simulink model "Sim2Twin_controlsystem_pos_Discrete"  (R2024b)
settings: Solver=FixedStepAuto  StartTime=0.0  StopTime=10.0  FixedStep=0.001  RelTol=1e-3
undefined symbols (not defined in the file): DiscIntNeverNeededParam, dspblkCoreblockFVToolHelper, gcbh
libraries: simulink x1
settings Model: Creator=Emila  LastModifiedBy=Are-Laptop
settings ConfigComp: PLC_OutputDir=XML  PLC_TargetIDE=twincat3  PLC_MultiTBSigbuilderTimeRange=off  PLC_FoldFBCallOutputVar=off  PLC_RemoveUnusedSSMethodCallArguments=off  PLC_UseCallOutputArgSyntax=off  PLC_EnableUnsignedAndDoubleTypes=off  PLC_EnableUDTSplitting=off  PLC_MaxFieldsInUDT=500  PLC_InlineEnumCastFunction=off

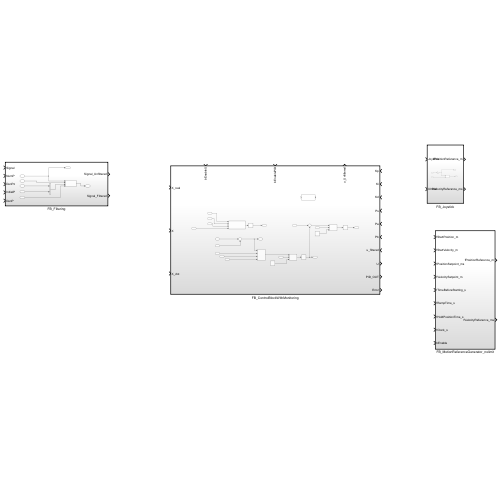
[thumbnail: Simulink's stored preview of the top-level diagram]
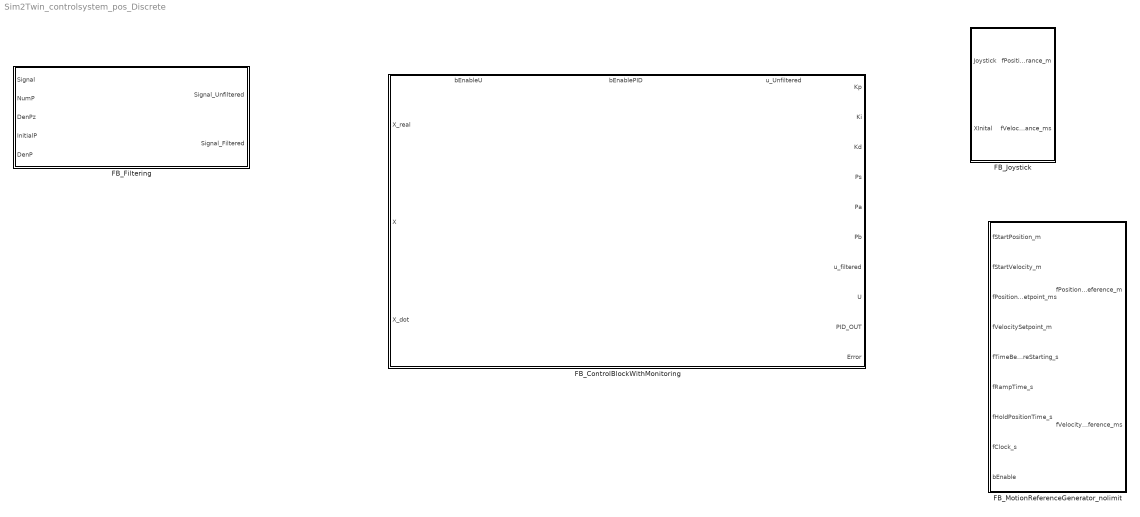
== system Sim2Twin_controlsystem_pos_Discrete ==
  FB_ControlBlockWithMonitoring : Subsystem  TreatAsAtomicUnit=on
      settings: PortSchema="{\"entries\":[{\"content\":{\"sides\":[{\"content\":{\"connectorIds\":[\"In1\",\"In2\",\"In3\"]},\"type\":\"ConnectorPlacement.EquallySpacedRectSide\",\"uuid\":\"e7dc98bc-0c39-42fc-9d44-5c528a861935\"},{\"content\":{\"connectorIds\":[\"In6\",\"In7\",\"In8\",\"In9\",\"In10\",\"In11\",\"In12\",\"Out1\",\"Out2\",\"Out3\"],\"side\":\"RIGHT\"},\"type\":\"ConnectorPlacement.EquallySpacedRectSide\",\"uuid\":\"7a7fb2e4-7f4e-4840-80a8-3a9723ecfbf6\"},{\"content\":{\"connectorIds\":[\"In4\",\"In5\",\"Out4\"],\"side\":\"TOP\"},\"type\":\"ConnectorPlacement.EquallySpacedRectSide\",\"uuid\":\"8314552e-40ce-493a-a910-ea6a3ee6c4fc\"},{\"content\":{\"side\":\"BOTTOM\"},\"type\":\"ConnectorPlacement.EquallySpacedRectSide\",\"uuid\":\"f3f01719-ff93-4fec-8599-54303ea6e608\"}]},\"type\":\"ConnectorPlacement.EquallySpacedConnector\",\"uuid\":\"904788e7-187d-4514-a00a-56ca1dbc298c\"}],\"packageUris\":[\"http://schema.mathworks.com/mf0/Connector/R2020b\"],\"version\":\"1.0\"}"
  FB_Filtering : Subsystem  TreatAsAtomicUnit=on
  FB_Joystick : Subsystem  TreatAsAtomicUnit=on
  FB_MotionReferenceGenerator_nolimit : Subsystem  TreatAsAtomicUnit=on  VariantControl=Ramp_Profile

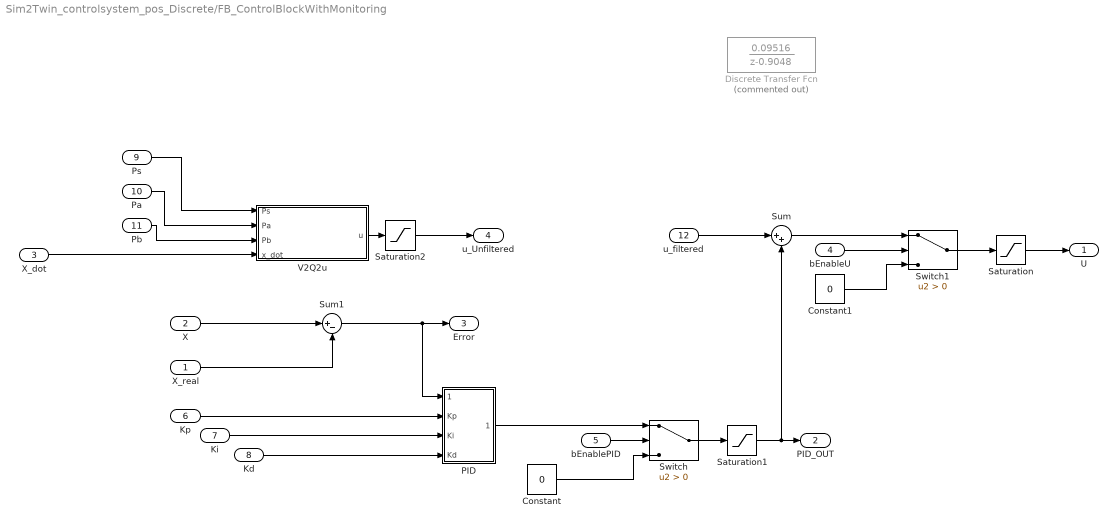
== system Sim2Twin_controlsystem_pos_Discrete/FB_ControlBlockWithMonitoring ==
  X_real : Inport
  X : Inport  Port=2
  X_dot : Inport  Port=3
  bEnableU : Inport  Port=4  OutDataTypeStr=boolean
  bEnablePID : Inport  Port=5  OutDataTypeStr=boolean
  Kp : Inport  Port=6
  Ki : Inport  Port=7
  Kd : Inport  Port=8
  Ps : Inport  Port=9
  Pa : Inport  Port=10
  Pb : Inport  Port=11
  u_filtered : Inport  Port=12
  Constant : Constant  Value=0
  Constant1 : Constant  Value=0
  Discrete Transfer Fcn : DiscreteTransferFcn  Commented=on  LoadFcn=dspblkCoreblockFVToolHelper(gcbh,'load');  Numerator=[0.09516]  Denominator=[1 -0.9048]
      settings: CopyFcn=dspblkCoreblockFVToolHelper(gcbh,'copy');  DeleteFcn=dspblkCoreblockFVToolHelper(gcbh,'close');  ModelCloseFcn=dspblkCoreblockFVToolHelper(gcbh,'close');  PreSaveFcn=dspblkCoreblockFVToolHelper(gcbh,'presave');  PostSaveFcn=dspblkCoreblockFVToolHelper(gcbh,'postsave');  CloseFcn=dspblkCoreblockFVToolHelper(gcbh,'close');
  PID : Subsystem
  Saturation : Saturate  UpperLimit=1  LowerLimit=-1
  Saturation1 : Saturate  UpperLimit=1  LowerLimit=-1
  Saturation2 : Saturate  UpperLimit=1  LowerLimit=-1
  Sum : Sum  Inputs=|++
  Sum1 : Sum  Inputs=|+-
  Switch : Switch  Criteria=u2 > Threshold  SaturateOnIntegerOverflow=off  InputSameDT=off
  Switch1 : Switch  Criteria=u2 > Threshold  SaturateOnIntegerOverflow=off  InputSameDT=off
  V2Q2u : MATLAB Function  TreatAsAtomicUnit=on
  U : Outport
  PID_OUT : Outport  Port=2
  Error : Outport  Port=3
  u_Unfiltered : Outport  Port=4
  wires:
  X_real/1 -> Sum1/2
  Sum1/1 -> Error/1, PID/1(PID_IN)
  V2Q2u/1(u) -> Saturation2/1
  X_dot/1 -> V2Q2u/4(x_dot)
  X/1 -> Sum1/1
  Switch/1 -> Saturation1/1
  PID/1(PID_OUT) -> Switch/1
  Switch1/1 -> Saturation/1
  Sum/1 -> Switch1/1
  bEnableU/1 -> Switch1/2
  bEnablePID/1 -> Switch/2
  Constant/1 -> Switch/3
  Constant1/1 -> Switch1/3
  Kp/1 -> PID/2(Kp)
  Ki/1 -> PID/3(Ki)
  Kd/1 -> PID/4(Kd)
  Saturation/1 -> U/1
  Saturation1/1 -> PID_OUT/1, Sum/2
  Saturation2/1 -> u_Unfiltered/1
  Pb/1 -> V2Q2u/3(Pb)
  Pa/1 -> V2Q2u/2(Pa)
  Ps/1 -> V2Q2u/1(Ps)
  u_filtered/1 -> Sum/1

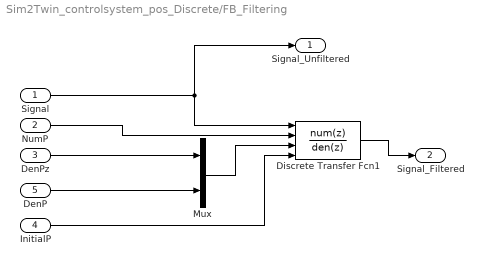
== system Sim2Twin_controlsystem_pos_Discrete/FB_Filtering ==
  Signal : Inport
  NumP : Inport  Port=2
  DenPz : Inport  Port=3
  InitialP : Inport  Port=4
  DenP : Inport  Port=5
  Discrete Transfer Fcn1 : DiscreteTransferFcn  LoadFcn=dspblkCoreblockFVToolHelper(gcbh,'load');  NumeratorSource=Input port  Numerator=[0.003137]  DenominatorSource=Input port  Denominator=[1 -0.9969]  InitialStatesSource=Input port  a0EqualsOne=on
      settings: CopyFcn=dspblkCoreblockFVToolHelper(gcbh,'copy');  DeleteFcn=dspblkCoreblockFVToolHelper(gcbh,'close');  ModelCloseFcn=dspblkCoreblockFVToolHelper(gcbh,'close');  PreSaveFcn=dspblkCoreblockFVToolHelper(gcbh,'presave');  PostSaveFcn=dspblkCoreblockFVToolHelper(gcbh,'postsave');  CloseFcn=dspblkCoreblockFVToolHelper(gcbh,'close');  InputPortMap=u0,p1,p3,p5
  Mux : Mux  Inputs=2
  Signal_Unfiltered : Outport
  Signal_Filtered : Outport  Port=2
  wires:
  InitialP/1 -> Discrete Transfer Fcn1/4
  DenP/1 -> Mux/2
  NumP/1 -> Discrete Transfer Fcn1/2
  DenPz/1 -> Mux/1
  Signal/1 -> Discrete Transfer Fcn1/1, Signal_Unfiltered/1
  Discrete Transfer Fcn1/1 -> Signal_Filtered/1
  Mux/1 -> Discrete Transfer Fcn1/3

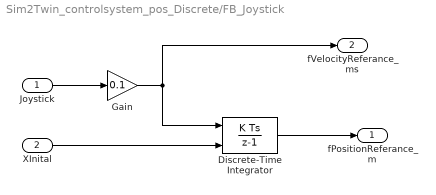
== system Sim2Twin_controlsystem_pos_Discrete/FB_Joystick ==
  Joystick : Inport
  XInital : Inport  Port=2
  Discrete-Time Integrator : DiscreteIntegrator  InitialConditionSource=external  SampleTime=-1  LimitOutput=on  UpperSaturationLimit=0.45  LowerSaturationLimit=0  ICPrevOutput=DiscIntNeverNeededParam  ICPrevScaledInput=DiscIntNeverNeededParam
  Gain : Gain  Gain=0.1
  fPositionReferance_m : Outport
  fVelocityReferance_ms : Outport  Port=2
  wires:
  Joystick/1 -> Gain/1
  Gain/1 -> Discrete-Time Integrator/1, fVelocityReferance_ms/1
  Discrete-Time Integrator/1 -> fPositionReferance_m/1
  XInital/1 -> Discrete-Time Integrator/2

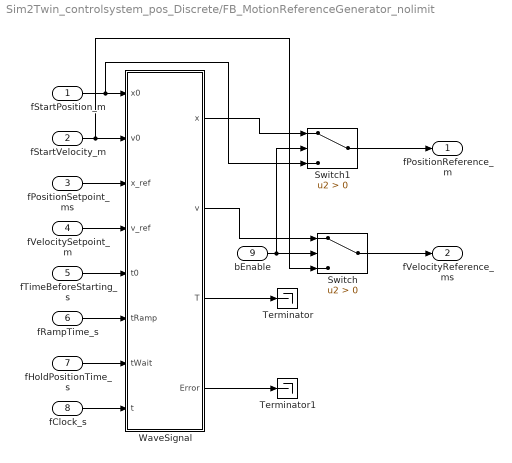
== system Sim2Twin_controlsystem_pos_Discrete/FB_MotionReferenceGenerator_nolimit ==
  fStartPosition_m : Inport
  fStartVelocity_m : Inport  Port=2
  fPositionSetpoint_ms : Inport  Port=3
  fVelocitySetpoint_m : Inport  Port=4
  fTimeBeforeStarting_s : Inport  Port=5
  fRampTime_s : Inport  Port=6
  fHoldPositionTime_s : Inport  Port=7
  fClock_s : Inport  Port=8
  bEnable : Inport  Port=9  OutDataTypeStr=boolean
  Switch : Switch  Criteria=u2 > Threshold  SaturateOnIntegerOverflow=off  InputSameDT=off
  Switch1 : Switch  Criteria=u2 > Threshold  SaturateOnIntegerOverflow=off  InputSameDT=off
  Terminator : Terminator
  Terminator1 : Terminator
  WaveSignal : MATLAB Function  TreatAsAtomicUnit=on
  fPositionReference_m : Outport  VectorParamsAs1DForOutWhenUnconnected=off
  fVelocityReference_ms : Outport  Port=2  VectorParamsAs1DForOutWhenUnconnected=off
  wires:
  fClock_s/1 -> WaveSignal/8(t)
  fTimeBeforeStarting_s/1 -> WaveSignal/5(t0)
  fPositionSetpoint_ms/1 -> WaveSignal/3(x_ref)
  fHoldPositionTime_s/1 -> WaveSignal/7(tWait)
  fVelocitySetpoint_m/1 -> WaveSignal/4(v_ref)
  WaveSignal/3(T) -> Terminator/1
  fRampTime_s/1 -> WaveSignal/6(tRamp)
  WaveSignal/4(Error) -> Terminator1/1
  WaveSignal/2(v) -> Switch/1
  fStartPosition_m/1 -> Switch1/3, WaveSignal/1(x0)
  Switch/1 -> fVelocityReference_ms/1
  bEnable/1 -> Switch1/2, Switch/2
  Switch1/1 -> fPositionReference_m/1
  WaveSignal/1(x) -> Switch1/1
  fStartVelocity_m/1 -> WaveSignal/2(v0), Switch/3

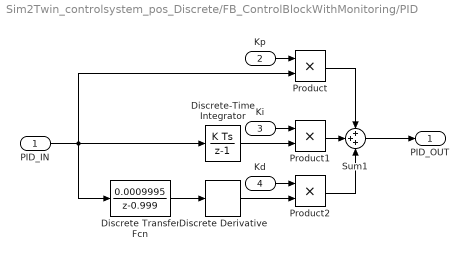
== system Sim2Twin_controlsystem_pos_Discrete/FB_ControlBlockWithMonitoring/PID ==
  PID_IN : Inport
  Kp : Inport  Port=2
  Ki : Inport  Port=3
  Kd : Inport  Port=4
  Discrete Transfer Fcn : DiscreteTransferFcn  LoadFcn=dspblkCoreblockFVToolHelper(gcbh,'load');  Numerator=[0.0009995]  Denominator=[1 -0.999]
      settings: CopyFcn=dspblkCoreblockFVToolHelper(gcbh,'copy');  DeleteFcn=dspblkCoreblockFVToolHelper(gcbh,'close');  ModelCloseFcn=dspblkCoreblockFVToolHelper(gcbh,'close');  PreSaveFcn=dspblkCoreblockFVToolHelper(gcbh,'presave');  PostSaveFcn=dspblkCoreblockFVToolHelper(gcbh,'postsave');  CloseFcn=dspblkCoreblockFVToolHelper(gcbh,'close');
  Discrete Derivative : simulink/Discrete/Discrete Derivative  gainval=1.0  ICPrevScaledInput=0.0  OutMin=[]  OutMax=[]  OutDataType=fixdt(1, 16)  OutScaling=2^-10  DoSatur=off
  Discrete-Time Integrator : DiscreteIntegrator  SampleTime=-1  ICPrevOutput=DiscIntNeverNeededParam  ICPrevScaledInput=DiscIntNeverNeededParam
  Product : Product
  Product1 : Product
  Product2 : Product
  Sum1 : Sum  Inputs=+++
  PID_OUT : Outport
  wires:
  Discrete Derivative/1 -> Product2/2
  Discrete-Time Integrator/1 -> Product1/2
  Product1/1 -> Sum1/2
  Product/1 -> Sum1/1
  PID_IN/1 -> Product/2, Discrete Transfer Fcn/1, Discrete-Time Integrator/1
  Product2/1 -> Sum1/3
  Sum1/1 -> PID_OUT/1
  Discrete Transfer Fcn/1 -> Discrete Derivative/1
  Kp/1 -> Product/1
  Ki/1 -> Product1/1
  Kd/1 -> Product2/1

== matlab function Sim2Twin_controlsystem_pos_Discrete/FB_MotionReferenceGenerator_nolimit/WaveSignal ==
  data: x0 input; v0 input; x_ref input; x output; v_ref input; t0 input; tRamp input; tWait input; v output; t input; T output; Error output double
function [x,v,T, Error] = fcn(x0,v0, x_ref,v_ref,t0,tRamp,tWait,t)
x_SP = x_ref - x0;
vs=v_ref;
slopeExt=v0-vs;
slopeRetr=-vs-v0;

as = vs/tRamp;
s_acc=(vs^2-v0^2)/as;

tHold=(x_SP-s_acc)/vs;

if tHold < 0
    Error = 1;
else
    Error = 0;
end

t1=tRamp;
t2=tHold;
t3=tRamp;
t4=tWait;
t5=t1;
t6=t2;
t7=t3;

x = x0;
x1 = x0 + v0*((t0+t1)-t0)-(slopeExt/t1)*((t0+t1)-t0)^2/2;
x2 = x1 + vs*((t0+t1+t2)-(t0+t1));
x4 = x_ref - v0*((t0+t1+t2+t3+t4+t5)-(t0+t1+t2+t3+t4))+(slopeRetr/t5)*((t0+t1+t2+t3+t4+t5)-(t0+t1+t2+t3+t4))^2/2;
x5 = x4-vs*((t0+t1+t2+t3+t4+t5+t6)-(t0+t1+t2+t3+t4+t5));

if Error == 1
    x = x0;
    v = v0;
elseif t>=0 && t<t0
    x = x0;
    v = v0;
elseif t>=t0 && t<(t0+t1)
    x = x0 + v0*(t-t0)-(slopeExt/t1)*(t-t0)^2/2;
    v = v0-(slopeExt/t1)*(t-t0);
elseif t>=(t0+t1) && t<(t0+t1+t2)
    x = x1 + vs*(t-(t0+t1));
    v = vs;
elseif t>=(t0+t1+t2) && t<(t0+t1+t2+t3)
    x = x2+vs*(t-(t0+t1+t2))+(slopeExt/t3)*(t-(t0+t1+t2))^2/2;
    v = vs+(slopeExt/t3)*(t-(t0+t1+t2));
elseif t>=(t0+t1+t2+t3) && t<(t0+t1+t2+t3+t4)
    x = x_ref;
    v = v0;
elseif t>=(t0+t1+t2+t3+t4) && t<(t0+t1+t2+t3+t4+t5)
    x = x_ref - v0*(t-(t0+t1+t2+t3+t4))+(slopeRetr/t5)*(t-(t0+t1+t2+t3+t4))^2/2;
    v = v0+(slopeRetr/t5)*(t-(t0+t1+t2+t3+t4));
elseif t>=(t0+t1+t2+t3+t4+t5) && t<(t0+t1+t2+t3+t4+t5+t6)
    x = x4-vs*(t-(t0+t1+t2+t3+t4+t5));
    v = -vs;
elseif t>=(t0+t1+t2+t3+t4+t5+t6) && t<(t0+t1+t2+t3+t4+t5+t6+t7)
    x = x5-vs*(t-(t0+t1+t2+t3+t4+t5+t6))-(slopeRetr/t3)*(t-(t0+t1+t2+t3+t4+t5+t6))^2/2;
    v = -vs-(slopeRetr/t3)*(t-(t0+t1+t2+t3+t4+t5+t6));
else
    x = x0;
    v = v0;
end

T = t0+t1+t2+t3+t4+t5+t6+t7;

== matlab function Sim2Twin_controlsystem_pos_Discrete/FB_ControlBlockWithMonitoring/V2Q2u ==
  data: Ps input; Pa input; Pb input; x_dot input; u output
function u = fcn(Ps, Pa, Pb, x_dot)

phi = 0.7130;
A = 33.1/100^2; % Area
BW = 0; % deadband
SpoolTravel = 7; % Maximum Spool Travel
a = (SpoolTravel-BW)/25; % Valve Slope Characteristic [mm/(L/min)]
dP_0 = 7e5; % Pressure drop with compansator

if x_dot > 0
    Q = x_dot * A; % Wanted Flow
    dP = (Ps-Pa)*1e5;
    dp_ref = abs(dP_0/dP);
    %dp_ref = 1;
    Q_star = (Q * sqrt(dp_ref)) * 6e4; % Referance Flow [L/min]
    u = (Q_star * a + BW)/SpoolTravel; % Control Signal [-1, 1]

elseif x_dot < 0
    Q = x_dot * (A*phi); % Wanted Flow
    dP = (Ps-Pb)*1e5;
    dp_ref = abs(dP_0/dP);
   % dp_ref = 1;
    Q_star = (Q * sqrt(dp_ref)) * 6e4; % Referance Flow [L/min]
    u = (Q_star * a - BW)/SpoolTravel; % Control Signal [-1, 1]

else
    u = 0;

end
end
